simulink library "I2tChecker"  (R2016b)
settings: Solver=VariableStepAuto  StartTime=0.0  StopTime=10.0  RelTol=1e-3
undefined symbols (not defined in the file): currentMaximum, currentNominal, currentTimeMaximum, thresholdI2tSurfaceWarning
settings Model: Creator=Nathan  LastModifiedBy=march

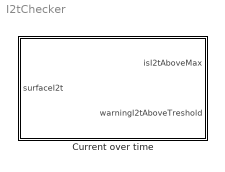
== system I2tChecker ==
  Current over time : Subsystem  ClipboardFcn=I2tLib

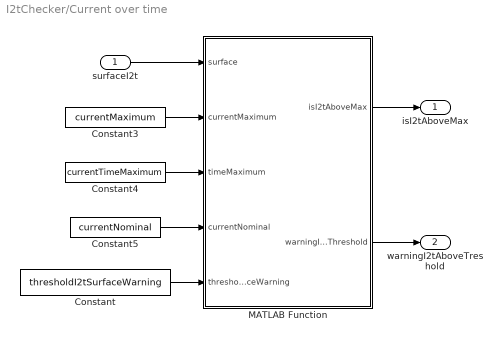
== system I2tChecker/Current over time ==
  surfaceI2t : Inport
  Constant : Constant  Value=thresholdI2tSurfaceWarning
  Constant3 : Constant  Value=currentMaximum  VectorParams1D=off  SampleTime=-1
  Constant4 : Constant  Value=currentTimeMaximum  VectorParams1D=off  SampleTime=-1
  Constant5 : Constant  Value=currentNominal  VectorParams1D=off  SampleTime=-1
  MATLAB Function : MATLAB Function  TreatAsAtomicUnit=on
  isI2tAboveMax : Outport  BusOutputAsStruct=on
  warningI2tAboveTreshold : Outport  Port=2
  wires:
  Constant/1 -> MATLAB Function/5(thresholdI2tSurfaceWarning)
  MATLAB Function/2(warningI2tAboveThreshold) -> warningI2tAboveTreshold/1
  MATLAB Function/1(isI2tAboveMax) -> isI2tAboveMax/1
  surfaceI2t/1 -> MATLAB Function/1(surface)
  Constant3/1 -> MATLAB Function/2(currentMaximum)
  Constant5/1 -> MATLAB Function/4(currentNominal)
  Constant4/1 -> MATLAB Function/3(timeMaximum)

== matlab function I2tChecker/Current over time/MATLAB Function ==
  data: surface input; isI2tAboveMax output; currentMaximum input; timeMaximum input; currentNominal input; warningI2tAboveThreshold output; thresholdI2tSurfaceWarning input
function [isI2tAboveMax,warningI2tAboveThreshold]  = fcn(surface, currentMaximum, timeMaximum, currentNominal, thresholdI2tSurfaceWarning)

% Initialize parameter
persistent prevError;
warningI2tAboveThreshold = 0;

% If the surface is still empty set it to 0
if isempty(prevError) 
    prevError = 0;
end

% The maximum I2t surface can be found
surfaceMaximum = timeMaximum * (currentMaximum^2 - currentNominal^2); %[I^2*t]

% Threshold for sending I2t warning
surfaceWarning = thresholdI2tSurfaceWarning*surfaceMaximum;

% Determine whether we are in a danger zone or not
if prevError == 0
    if surface > surfaceMaximum
        isI2tAboveMax = 1;
    else
        isI2tAboveMax = 0;
    end
else
    if surface > 0.5 * surfaceMaximum
        isI2tAboveMax = 1;
    else
        isI2tAboveMax = 0;
    end
end

if ((surface > surfaceWarning) && isI2tAboveMax ~= 1)
    warningI2tAboveThreshold = 1;
else
    warningI2tAboveThreshold = 0;
end

% update persistent variables
prevError = isI2tAboveMax;
end
